simulink model "Lab"  (R2022b)
settings: Solver=VariableStepAuto  StartTime=0.0  StopTime=15  RelTol=1e-3
settings Model: Creator=ahmed  LastModifiedBy=ahmed

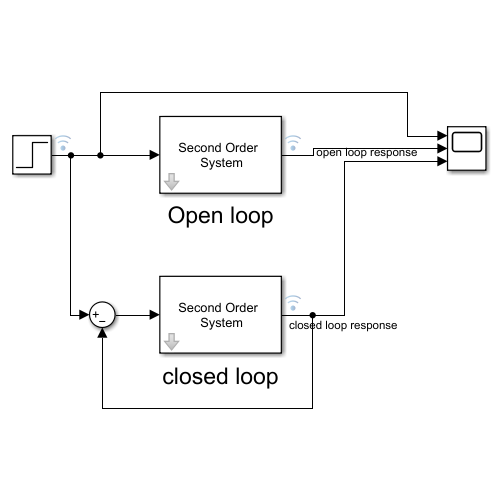
[thumbnail: Simulink's stored preview of the top-level diagram]
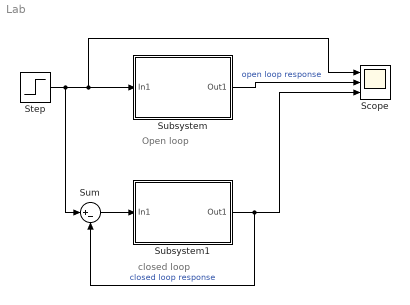
== system Lab ==
  note: Open loop
  note: closed loop
  Scope : Scope  NumInputPorts=3
  Step : Step  SampleTime=0
  Subsystem : Subsystem  mask{zeta=0.7, wn=1}
      mask prompts: zeta "Damping ratio"; wn "Natural Frequancy"
      mask DialogControl DescGroupVar Prompt: Second order
      mask DialogControl DescTextVar Prompt: this block simulate second order transfer function equation
      mask Display: disp('Second Order \n System');
  Subsystem1 : Subsystem  mask{zeta=0.7, wn=1}
      mask prompts: zeta "Damping ratio"; wn "Natural Frequancy"
      mask DialogControl DescGroupVar Prompt: Second order
      mask DialogControl DescTextVar Prompt: this block simulate second order transfer function equation
      mask Display: disp('Second Order \n System');
  Sum : Sum  Inputs=|+-
  wires:
  Step/1 -> Sum/1, Scope/1, Subsystem/1(In1)
  Subsystem/1(Out1) -> Scope/2  "open loop response"
  Subsystem1/1(Out1) -> Scope/3, Sum/2  "closed loop response"
  Sum/1 -> Subsystem1/1(In1)

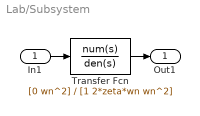
== system Lab/Subsystem ==
  In1 : Inport
  Transfer Fcn : TransferFcn  Numerator=[0 wn^2]  Denominator=[1 2*zeta*wn wn^2]
  Out1 : Outport
  wires:
  In1/1 -> Transfer Fcn/1
  Transfer Fcn/1 -> Out1/1

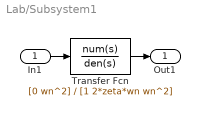
== system Lab/Subsystem1 ==
  In1 : Inport
  Transfer Fcn : TransferFcn  Numerator=[0 wn^2]  Denominator=[1 2*zeta*wn wn^2]
  Out1 : Outport
  wires:
  Transfer Fcn/1 -> Out1/1
  In1/1 -> Transfer Fcn/1
